simulink model "mconversion5"  (Simulink 8.0)
settings: Solver=FixedStepDiscrete  StartTime=0.0  StopTime=10.0  RelTol=1e-3
settings Model: Creator=awarlock  LastModifiedBy=htu  ExtModeAutoUpdateStatusClock=off
settings DataIOCC: SignalLoggingSaveFormat=ModelDataLogs  SaveOutput=off  SaveTime=off  SignalLoggingName=logsOut
settings OptimizationCC: InlineParams=on  InlineInvariantSignals=on  InitFltsAndDblsToZero=on
settings DebuggingCC: SaveWithParameterizedLinksMsg=none  CheckExecutionContextPreStartOutputMsg=on  CheckExecutionContextRuntimeOutputMsg=on  SignalResolutionControl=TryResolveAllWithWarning  MultiTaskDSMMsg=warning  MultiTaskCondExecSysMsg=none
settings RTWCC: IncludeERTFirstTime=on
settings GRTTargetCC: TargetFcnLib=ansi_tfl_tmw.mat  CombineOutputUpdateFcns=off  GRTInterface=on

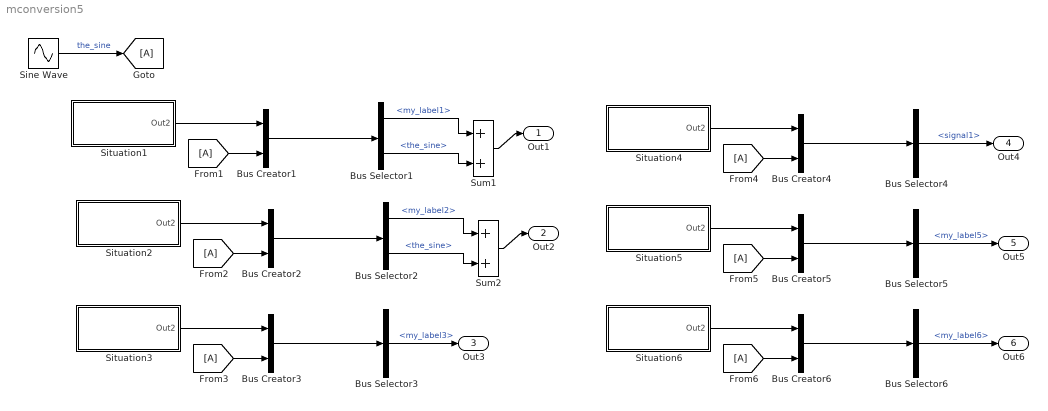
== system mconversion5 ==
  Bus Creator{1..6} (6 alike) : BusCreator  DialogController=Simulink.DDGSource_Bus  Inputs=2
  Bus Selector1 : BusSelector  DialogController=Simulink.DDGSource_Bus  OutputSignals=my_label1,the_sine
  Bus Selector2 : BusSelector  DialogController=Simulink.DDGSource_Bus  OutputSignals=my_label2,the_sine
  Bus Selector3 : BusSelector  DialogController=Simulink.DDGSource_Bus  OutputSignals=my_label3
  Bus Selector4 : BusSelector  DialogController=Simulink.DDGSource_Bus  OutputSignals=signal1
  Bus Selector5 : BusSelector  DialogController=Simulink.DDGSource_Bus  OutputSignals=my_label5
  Bus Selector6 : BusSelector  DialogController=Simulink.DDGSource_Bus  OutputSignals=my_label6
  Sine Wave : Sin  SampleTime=0.1
  Situation1 : Subsystem  TreatAsAtomicUnit=on
  Situation2 : Subsystem  TreatAsAtomicUnit=on
  Situation3 : Subsystem  TreatAsAtomicUnit=on
  Situation4 : Subsystem  TreatAsAtomicUnit=on
  Situation5 : Subsystem  TreatAsAtomicUnit=on
  Situation6 : Subsystem  TreatAsAtomicUnit=on
  Sum1 : Sum  Inputs=|++
  Sum2 : Sum  Inputs=|++
  Out1 : Outport
  Out2 : Outport  Port=2
  Out3 : Outport  Port=3
  Out4 : Outport  Port=4
  Out5 : Outport  Port=5
  Out6 : Outport  Port=6
  wires:
  Situation1/1(Out2) -> Bus Creator1/1
  Bus Creator1/1 -> Bus Selector1/1
  Sine Wave/1 -> [A]  "the_sine"
  [A] -> Bus Creator1/2
  Bus Selector1/1 -> Sum1/1  "<my_label1>"
  Bus Selector1/2 -> Sum1/2  "<the_sine>"
  Sum1/1 -> Out1/1
  Situation2/1(Out2) -> Bus Creator2/1
  Bus Creator2/1 -> Bus Selector2/1
  [A] -> Bus Creator2/2
  Bus Selector2/1 -> Sum2/1  "<my_label2>"
  Bus Selector2/2 -> Sum2/2  "<the_sine>"
  Sum2/1 -> Out2/1
  Situation3/1(Out2) -> Bus Creator3/1
  Bus Creator3/1 -> Bus Selector3/1
  [A] -> Bus Creator3/2
  Situation4/1(Out2) -> Bus Creator4/1
  Bus Creator4/1 -> Bus Selector4/1
  [A] -> Bus Creator4/2
  Situation5/1(Out2) -> Bus Creator5/1
  Bus Creator5/1 -> Bus Selector5/1
  [A] -> Bus Creator5/2
  Situation6/1(Out2) -> Bus Creator6/1
  Bus Creator6/1 -> Bus Selector6/1
  [A] -> Bus Creator6/2
  Bus Selector3/1 -> Out3/1  "<my_label3>"
  Bus Selector4/1 -> Out4/1  "<signal1>"
  Bus Selector5/1 -> Out5/1  "<my_label5>"
  Bus Selector6/1 -> Out6/1  "<my_label6>"

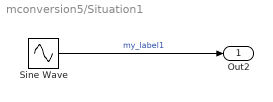
== system mconversion5/Situation1 ==
  Sine Wave : Sin  SampleTime=0.1
  Out2 : Outport
  wires:
  Sine Wave/1 -> Out2/1  "my_label1"

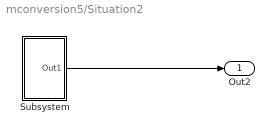
== system mconversion5/Situation2 ==
  Subsystem : Subsystem
  Out2 : Outport
  wires:
  Subsystem/1(Out1) -> Out2/1

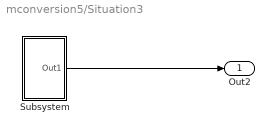
== system mconversion5/Situation3 ==
  Subsystem : Subsystem
  Out2 : Outport
  wires:
  Subsystem/1(Out1) -> Out2/1

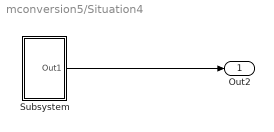
== system mconversion5/Situation4 ==
  Subsystem : Subsystem
  Out2 : Outport
  wires:
  Subsystem/1(Out1) -> Out2/1

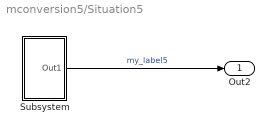
== system mconversion5/Situation5 ==
  Subsystem : Subsystem
  Out2 : Outport
  wires:
  Subsystem/1(Out1) -> Out2/1  "my_label5"

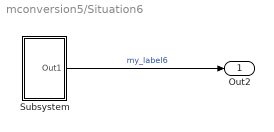
== system mconversion5/Situation6 ==
  Subsystem : Subsystem
  Out2 : Outport
  wires:
  Subsystem/1(Out1) -> Out2/1  "my_label6"

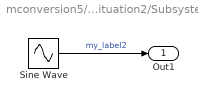
== system mconversion5/Situation2/Subsystem ==
  Sine Wave : Sin  SampleTime=0.1
  Out1 : Outport
  wires:
  Sine Wave/1 -> Out1/1  "my_label2"

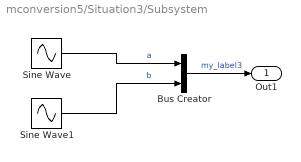
== system mconversion5/Situation3/Subsystem ==
  Bus Creator : BusCreator  DialogController=Simulink.DDGSource_Bus  Inputs=2
  Sine Wave : Sin  SampleTime=0.1
  Sine Wave1 : Sin  SampleTime=0.1
  Out1 : Outport
  wires:
  Sine Wave/1 -> Bus Creator/1  "a"
  Bus Creator/1 -> Out1/1  "my_label3"
  Sine Wave1/1 -> Bus Creator/2  "b"

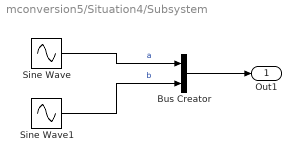
== system mconversion5/Situation4/Subsystem ==
  Bus Creator : BusCreator  DialogController=Simulink.DDGSource_Bus  Inputs=2
  Sine Wave : Sin  SampleTime=0.1
  Sine Wave1 : Sin  SampleTime=0.1
  Out1 : Outport
  wires:
  Sine Wave1/1 -> Bus Creator/2  "b"
  Bus Creator/1 -> Out1/1
  Sine Wave/1 -> Bus Creator/1  "a"

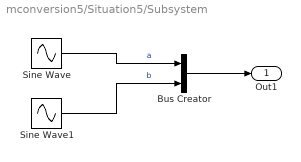
== system mconversion5/Situation5/Subsystem ==
  Bus Creator : BusCreator  DialogController=Simulink.DDGSource_Bus  Inputs=2
  Sine Wave : Sin  SampleTime=0.1
  Sine Wave1 : Sin  SampleTime=0.1
  Out1 : Outport
  wires:
  Sine Wave/1 -> Bus Creator/1  "a"
  Bus Creator/1 -> Out1/1
  Sine Wave1/1 -> Bus Creator/2  "b"

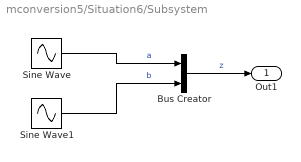
== system mconversion5/Situation6/Subsystem ==
  Bus Creator : BusCreator  DialogController=Simulink.DDGSource_Bus  Inputs=2
  Sine Wave : Sin  SampleTime=0.1
  Sine Wave1 : Sin  SampleTime=0.1
  Out1 : Outport
  wires:
  Sine Wave1/1 -> Bus Creator/2  "b"
  Bus Creator/1 -> Out1/1  "z"
  Sine Wave/1 -> Bus Creator/1  "a"
